simulink model "altitude_controller"  (R2025b)
settings: Solver=FixedStepAuto  StartTime=0.0  StopTime=inf  FixedStep=0.1  RelTol=1e-3
libraries: slpidlib x3, instrumentlib x2, uavutilslib x1
settings Model: Creator=Rakshan  LastModifiedBy=Rakshan

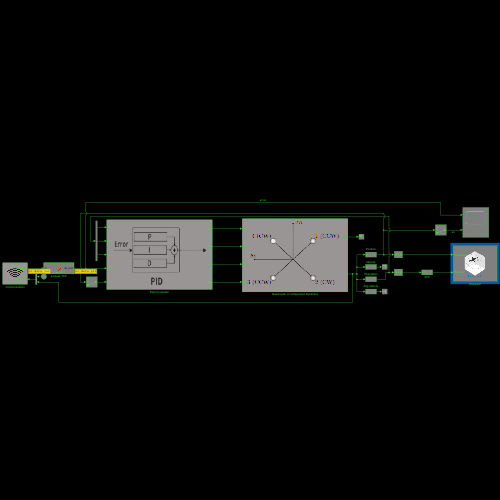
[thumbnail: Simulink's stored preview of the top-level diagram]
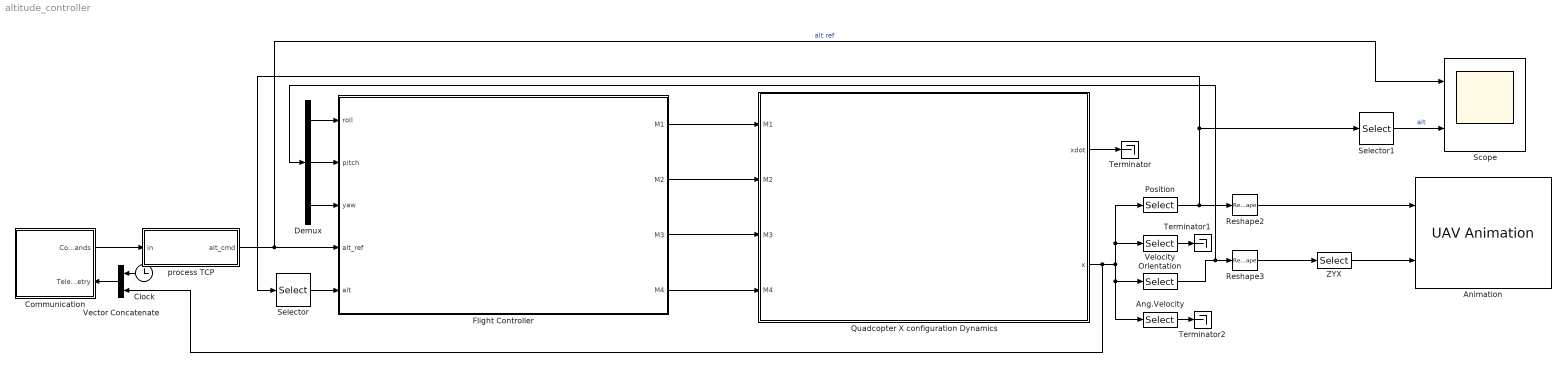
== system altitude_controller ==
  Ang.Velocity : Selector  InputPortWidth=12  IndexOptions=Index vector (dialog)  Indices=[10 11 12]  OutputSizes=1
  Animation : uavutilslib/UAV Animation  NumUAV=1  DynamicUAVConfig=off  UAVType=Multirotor  UAVSize=1  UAVColor=[1, 0.8, 0]  UAVTrajectoryAlpha=1  InertialZDirection=Up  RotationFormat=Euler ZYX  DrawMarkers=off  SampleTime=-1
  Clock : Clock
  Communication : Subsystem
      settings: PortSchema="{\"entries\":[{\"content\":{\"sides\":[{\"content\":{},\"type\":\"ConnectorPlacement.EquallySpacedRectSide\",\"uuid\":\"c4d22659-2383-4074-b14f-30b672d720eb\"},{\"content\":{\"connectorIds\":[\"Out1\",\"In1\"],\"side\":\"RIGHT\"},\"type\":\"ConnectorPlacement.EquallySpacedRectSide\",\"uuid\":\"ba8f1d3a-a611-4235-8c7a-b63cea4c0df4\"},{\"content\":{\"side\":\"TOP\"},\"type\":\"ConnectorPlacement.EquallySpacedRectSide\",\"uuid\":\"69655158-725a-45bc-a08c-7abd09db6858\"}]},\"type\":\"ConnectorPlacement.EquallySpacedConnector\",\"uuid\":\"62f793ea-cbc8-4bf1-b4ec-cf6c7e8acac7\"}],\"packageUris\":[\"http://schema.mathworks.com/mf0/Connector/R2020b\"],\"version\":\"1.0\"}"
      mask Display: image('communication-Photoroom.png');
  Demux : Demux  Outputs=3
  Flight Controller : Subsystem
      mask Display: image('pid-Photoroom.png');
  Orientation : Selector  InputPortWidth=12  IndexOptions=Index vector (dialog)  Indices=[7 8 9]  OutputSizes=1
  Position : Selector  InputPortWidth=12  IndexOptions=Index vector (dialog)  Indices=[1 2 3]  OutputSizes=1
  Quadcopter X configuration Dynamics : Subsystem
      mask Display: image('axis-Photoroom.png');
  Reshape2 : Reshape  OutputDimensionality=Row vector (2-D)
  Reshape3 : Reshape  OutputDimensionality=Row vector (2-D)
  Scope : Scope  NumInputPorts=2
      settings: ActiveDisplayYMinimum=-3.2874736842437113  ActiveDisplayYMaximum=28.143052631582634
  Selector : Selector  InputPortWidth=3  IndexOptions=Index vector (dialog)  Indices=3  OutputSizes=1
  Selector1 : Selector  InputPortWidth=3  IndexOptions=Index vector (dialog)  Indices=3  OutputSizes=1
  Terminator : Terminator
  Terminator1 : Terminator
  Terminator2 : Terminator
  Vector Concatenate : Concatenate
  Velocity : Selector  InputPortWidth=12  IndexOptions=Index vector (dialog)  Indices=[4 5 6]  OutputSizes=1
  ZYX : Selector  InputPortWidth=3  IndexOptions=Index vector (dialog)  Indices=[3 2 1]  OutputSizes=1
  process TCP : MATLAB Function  TreatAsAtomicUnit=on
  wires:
  Communication/1(Commands) -> process TCP/1(in)
  Flight Controller/2(M2) -> Quadcopter X configuration Dynamics/2(M2)
  Flight Controller/1(M1) -> Quadcopter X configuration Dynamics/1(M1)
  Flight Controller/3(M3) -> Quadcopter X configuration Dynamics/3(M3)
  Flight Controller/4(M4) -> Quadcopter X configuration Dynamics/4(M4)
  Quadcopter X configuration Dynamics/1(xdot) -> Terminator/1
  Position/1 -> Selector1/1, Selector/1, Reshape2/1
  Orientation/1 -> Demux/1, Reshape3/1
  Velocity/1 -> Terminator1/1
  Ang.Velocity/1 -> Terminator2/1
  Reshape2/1 -> Animation/1
  Reshape3/1 -> ZYX/1
  ZYX/1 -> Animation/2
  process TCP/1(alt_cmd) -> Scope/1, Flight Controller/4(alt_ref)  "alt ref"
  Demux/1 -> Flight Controller/1(roll)
  Demux/2 -> Flight Controller/2(pitch)
  Demux/3 -> Flight Controller/3(yaw)
  Selector/1 -> Flight Controller/5(alt)
  Selector1/1 -> Scope/2  "alt"
  Quadcopter X configuration Dynamics/2(x) -> Vector Concatenate/2, Orientation/1, Ang.Velocity/1, Position/1, Velocity/1
  Clock/1 -> Vector Concatenate/1
  Vector Concatenate/1 -> Communication/1(Telemetry)

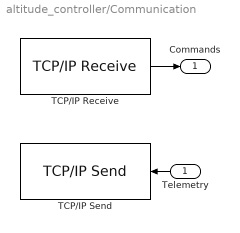
== system altitude_controller/Communication ==
  Telemetry : Inport
  TCP/IP Receive : instrumentlib/TCP//IP Receive  Host=127.0.0.1  Port=55000  DataSize=[ 1, 2 ]  DataType=double  ASCIIFormatting=%f  Terminator=LF  CustomTerminator=10  ByteOrder=big-endian  EnableBlockingMode=on  Timeout=1  SampleTime=0.1  SimulateUsing=Interpreted execution
  TCP/IP Send : instrumentlib/TCP//IP Send  Host=127.0.0.1  Port=55001  ByteOrder=big-endian  EnableBlockingMode=off  Timeout=10  TransferDelay=on  SimulateUsing=Interpreted execution
  Commands : Outport
  wires:
  TCP/IP Receive/1 -> Commands/1
  Telemetry/1 -> TCP/IP Send/1

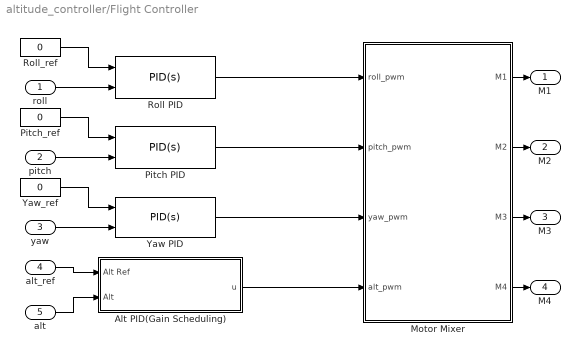
== system altitude_controller/Flight Controller ==
  roll : Inport
  pitch : Inport  Port=2
  yaw : Inport  Port=3
  alt_ref : Inport  Port=4
  alt : Inport  Port=5
  Alt PID(Gain Scheduling) : Subsystem
  Motor Mixer : MATLAB Function  TreatAsAtomicUnit=on
  Pitch PID : slpidlib/PID Controller (2DOF)  Controller=PID  Form=Parallel  TimeDomain=Continuous-time  UseExternalTs=off  SampleTime=-1  IntegratorMethod=Forward Euler  FilterMethod=Forward Euler  ControllerParametersSource=internal  P=1  I=0  UseKiTs=off  D=0  UseExternalDerivativeSource=off  N=100  UseFilter=on  b=1  c=1  TunerSelectOption=Transfer Function Based (PID Tuner App)  InitialConditionSource=internal  InitialConditionForIntegrator=0  InitialConditionForFilter=0  DifferentiatorICPrevScaledInput=0  ExternalReset=none  TrackingMode=off  Kt=1  LimitOutput=off  SatLimitsSource=internal  UpperSaturationLimit=inf  LowerSaturationLimit=-inf  LinearizeAsGain=on  AntiWindupMode=none  Kb=1  LimitIntegrator=off  UpperIntegratorSaturationLimit=inf  LowerIntegratorSaturationLimit=-inf  POutMin=[]  POutMax=[]  IOutMin=[]  IOutMax=[]  DOutMin=[]  DOutMax=[]  NOutMin=[]  NOutMax=[]  bOutMin=[]  bOutMax=[]  cOutMin=[]  cOutMax=[]  SumOutMin=[]  SumOutMax=[]  SaturationOutMin=[]  SaturationOutMax=[]  PParamMin=[]  PParamMax=[]  IParamMin=[]  IParamMax=[]  DParamMin=[]  DParamMax=[]  NParamMin=[]  NParamMax=[]  bParamMin=[]  bParamMax=[]  cParamMin=[]  cParamMax=[]  KbParamMin=[]  KbParamMax=[]  KtParamMin=[]  KtParamMax=[]  KbOutMin=[]  KbOutMax=[]  KtOutMin=[]  KtOutMax=[]  IntegratorOutMin=[]  IntegratorOutMax=[]  FilterOutMin=[]  FilterOutMax=[]  SumI1OutMin=[]  SumI1OutMax=[]  SumI2OutMin=[]  SumI2OutMax=[]  SumI3OutMin=[]  SumI3OutMax=[]  SumI4OutMin=[]  SumI4OutMax=[]  SumDOutMin=[]  SumDOutMax=[]  Sum1OutMin=[]  Sum1OutMax=[]  Sum2OutMin=[]  Sum2OutMax=[]  Sum3OutMin=[]  Sum3OutMax=[]  DifferentiatorOutMin=[]  DifferentiatorOutMax=[]  FilterDiffOutCoefMin=[]  FilterDiffOutCoefMax=[]  ReciprocalOutMin=[]  ReciprocalOutMax=[]  SumDenOutMin=[]  SumDenOutMax=[]  SumNumOutMin=[]  SumNumOutMax=[]  DivideOutMin=[]  DivideOutMax=[]  UdiffTsProdOutMin=[]  UdiffTsProdOutMax=[]  NTsProdOutMin=[]  NTsProdOutMax=[]  UintegralTsProdOutMin=[]  UintegralTsProdOutMax=[]  UngainTsProdOutMin=[]  UngainTsProdOutMax=[]  ClampingZeroOutDataTypeStr=Inherit: Inherit via back propagation  ClampingZeroOutMin=[]  ClampingZeroOutMax=[]  FilterDenConstantOutDataTypeStr=Inherit: Inherit via back propagation  FilterDenConstantOutMin=[]  FilterDenConstantOutMax=[]  PCopyOutDataTypeStr=Inherit: Inherit via back propagation  PCopyOutMin=[]  PCopyOutMax=[]  NCopyOutDataTypeStr=Inherit: Inherit via back propagation  NCopyOutMin=[]  NCopyOutMax=[]  IntegratorContinuousStateAttributes=''  IntegratorStateMustResolveToSignalObject=off  IntegratorRTWStateStorageClass=Auto  FilterContinuousStateAttributes=''  FilterStateMustResolveToSignalObject=off  FilterRTWStateStorageClass=Auto  ParallelPVariant=InternalParameters  IdealPVariant=Disabled  IVariant=InternalParameters  DVariant=InternalParameters  bVariant=InternalParameters  cVariant=InternalParameters  IntegratorVariant=Continuous  SatVariant=Disabled  AWVariant=Passthrough  PCopyVariant=Disabled  TRVariant=Disabled  FdbkBlocksVariant=Forward  IdealPFdbkVariant=Disabled  SatFdbkVariant=Disabled  DerivativeFilterVariant=ContFilter  NVariant=InternalParameters  NCopyVariant=Disabled  FilterICVariant=InternalICsFilter  IntegratorICVariant=InternalICs  ExternalResetVariant=Disabled  TRSumVariant=Passthrough  SumFdbkVariant=Disabled  SumVariant=Sum_PID  TsampFilterVariant=InternalTs  TsampNgainVariant=Passthrough  TsampIntegralVariant=Disabled_SignalSpec  ExternalSaturationOutDataTypeStr=Inherit: Same as second input  DerivativeSourceVariant=ErrorSignal  PreIntVariant=InternalPreInt
  Pitch_ref : Constant  Value=0
  Roll PID : slpidlib/PID Controller (2DOF)  Controller=PID  Form=Parallel  TimeDomain=Continuous-time  UseExternalTs=off  SampleTime=-1  IntegratorMethod=Forward Euler  FilterMethod=Forward Euler  ControllerParametersSource=internal  P=1  I=0  UseKiTs=off  D=0.1  UseExternalDerivativeSource=off  N=100  UseFilter=on  b=1  c=1  TunerSelectOption=Transfer Function Based (PID Tuner App)  InitialConditionSource=internal  InitialConditionForIntegrator=0  InitialConditionForFilter=0  DifferentiatorICPrevScaledInput=0  ExternalReset=none  TrackingMode=off  Kt=1  LimitOutput=off  SatLimitsSource=internal  UpperSaturationLimit=inf  LowerSaturationLimit=-inf  LinearizeAsGain=on  AntiWindupMode=none  Kb=1  LimitIntegrator=off  UpperIntegratorSaturationLimit=inf  LowerIntegratorSaturationLimit=-inf  POutMin=[]  POutMax=[]  IOutMin=[]  IOutMax=[]  DOutMin=[]  DOutMax=[]  NOutMin=[]  NOutMax=[]  bOutMin=[]  bOutMax=[]  cOutMin=[]  cOutMax=[]  SumOutMin=[]  SumOutMax=[]  SaturationOutMin=[]  SaturationOutMax=[]  PParamMin=[]  PParamMax=[]  IParamMin=[]  IParamMax=[]  DParamMin=[]  DParamMax=[]  NParamMin=[]  NParamMax=[]  bParamMin=[]  bParamMax=[]  cParamMin=[]  cParamMax=[]  KbParamMin=[]  KbParamMax=[]  KtParamMin=[]  KtParamMax=[]  KbOutMin=[]  KbOutMax=[]  KtOutMin=[]  KtOutMax=[]  IntegratorOutMin=[]  IntegratorOutMax=[]  FilterOutMin=[]  FilterOutMax=[]  SumI1OutMin=[]  SumI1OutMax=[]  SumI2OutMin=[]  SumI2OutMax=[]  SumI3OutMin=[]  SumI3OutMax=[]  SumI4OutMin=[]  SumI4OutMax=[]  SumDOutMin=[]  SumDOutMax=[]  Sum1OutMin=[]  Sum1OutMax=[]  Sum2OutMin=[]  Sum2OutMax=[]  Sum3OutMin=[]  Sum3OutMax=[]  DifferentiatorOutMin=[]  DifferentiatorOutMax=[]  FilterDiffOutCoefMin=[]  FilterDiffOutCoefMax=[]  ReciprocalOutMin=[]  ReciprocalOutMax=[]  SumDenOutMin=[]  SumDenOutMax=[]  SumNumOutMin=[]  SumNumOutMax=[]  DivideOutMin=[]  DivideOutMax=[]  UdiffTsProdOutMin=[]  UdiffTsProdOutMax=[]  NTsProdOutMin=[]  NTsProdOutMax=[]  UintegralTsProdOutMin=[]  UintegralTsProdOutMax=[]  UngainTsProdOutMin=[]  UngainTsProdOutMax=[]  ClampingZeroOutDataTypeStr=Inherit: Inherit via back propagation  ClampingZeroOutMin=[]  ClampingZeroOutMax=[]  FilterDenConstantOutDataTypeStr=Inherit: Inherit via back propagation  FilterDenConstantOutMin=[]  FilterDenConstantOutMax=[]  PCopyOutDataTypeStr=Inherit: Inherit via back propagation  PCopyOutMin=[]  PCopyOutMax=[]  NCopyOutDataTypeStr=Inherit: Inherit via back propagation  NCopyOutMin=[]  NCopyOutMax=[]  IntegratorContinuousStateAttributes=''  IntegratorStateMustResolveToSignalObject=off  IntegratorRTWStateStorageClass=Auto  FilterContinuousStateAttributes=''  FilterStateMustResolveToSignalObject=off  FilterRTWStateStorageClass=Auto  ParallelPVariant=InternalParameters  IdealPVariant=Disabled  IVariant=InternalParameters  DVariant=InternalParameters  bVariant=InternalParameters  cVariant=InternalParameters  IntegratorVariant=Continuous  SatVariant=Disabled  AWVariant=Passthrough  PCopyVariant=Disabled  TRVariant=Disabled  FdbkBlocksVariant=Forward  IdealPFdbkVariant=Disabled  SatFdbkVariant=Disabled  DerivativeFilterVariant=ContFilter  NVariant=InternalParameters  NCopyVariant=Disabled  FilterICVariant=InternalICsFilter  IntegratorICVariant=InternalICs  ExternalResetVariant=Disabled  TRSumVariant=Passthrough  SumFdbkVariant=Disabled  SumVariant=Sum_PID  TsampFilterVariant=InternalTs  TsampNgainVariant=Passthrough  TsampIntegralVariant=Disabled_SignalSpec  ExternalSaturationOutDataTypeStr=Inherit: Same as second input  DerivativeSourceVariant=ErrorSignal  PreIntVariant=InternalPreInt
  Roll_ref : Constant  Value=0
  Yaw PID : slpidlib/PID Controller (2DOF)  Controller=PID  Form=Parallel  TimeDomain=Continuous-time  UseExternalTs=off  SampleTime=-1  IntegratorMethod=Forward Euler  FilterMethod=Forward Euler  ControllerParametersSource=internal  P=1  I=0  UseKiTs=off  D=0  UseExternalDerivativeSource=off  N=100  UseFilter=on  b=1  c=1  TunerSelectOption=Transfer Function Based (PID Tuner App)  InitialConditionSource=internal  InitialConditionForIntegrator=0  InitialConditionForFilter=0  DifferentiatorICPrevScaledInput=0  ExternalReset=none  TrackingMode=off  Kt=1  LimitOutput=off  SatLimitsSource=internal  UpperSaturationLimit=inf  LowerSaturationLimit=-inf  LinearizeAsGain=on  AntiWindupMode=none  Kb=1  LimitIntegrator=off  UpperIntegratorSaturationLimit=inf  LowerIntegratorSaturationLimit=-inf  POutMin=[]  POutMax=[]  IOutMin=[]  IOutMax=[]  DOutMin=[]  DOutMax=[]  NOutMin=[]  NOutMax=[]  bOutMin=[]  bOutMax=[]  cOutMin=[]  cOutMax=[]  SumOutMin=[]  SumOutMax=[]  SaturationOutMin=[]  SaturationOutMax=[]  PParamMin=[]  PParamMax=[]  IParamMin=[]  IParamMax=[]  DParamMin=[]  DParamMax=[]  NParamMin=[]  NParamMax=[]  bParamMin=[]  bParamMax=[]  cParamMin=[]  cParamMax=[]  KbParamMin=[]  KbParamMax=[]  KtParamMin=[]  KtParamMax=[]  KbOutMin=[]  KbOutMax=[]  KtOutMin=[]  KtOutMax=[]  IntegratorOutMin=[]  IntegratorOutMax=[]  FilterOutMin=[]  FilterOutMax=[]  SumI1OutMin=[]  SumI1OutMax=[]  SumI2OutMin=[]  SumI2OutMax=[]  SumI3OutMin=[]  SumI3OutMax=[]  SumI4OutMin=[]  SumI4OutMax=[]  SumDOutMin=[]  SumDOutMax=[]  Sum1OutMin=[]  Sum1OutMax=[]  Sum2OutMin=[]  Sum2OutMax=[]  Sum3OutMin=[]  Sum3OutMax=[]  DifferentiatorOutMin=[]  DifferentiatorOutMax=[]  FilterDiffOutCoefMin=[]  FilterDiffOutCoefMax=[]  ReciprocalOutMin=[]  ReciprocalOutMax=[]  SumDenOutMin=[]  SumDenOutMax=[]  SumNumOutMin=[]  SumNumOutMax=[]  DivideOutMin=[]  DivideOutMax=[]  UdiffTsProdOutMin=[]  UdiffTsProdOutMax=[]  NTsProdOutMin=[]  NTsProdOutMax=[]  UintegralTsProdOutMin=[]  UintegralTsProdOutMax=[]  UngainTsProdOutMin=[]  UngainTsProdOutMax=[]  ClampingZeroOutDataTypeStr=Inherit: Inherit via back propagation  ClampingZeroOutMin=[]  ClampingZeroOutMax=[]  FilterDenConstantOutDataTypeStr=Inherit: Inherit via back propagation  FilterDenConstantOutMin=[]  FilterDenConstantOutMax=[]  PCopyOutDataTypeStr=Inherit: Inherit via back propagation  PCopyOutMin=[]  PCopyOutMax=[]  NCopyOutDataTypeStr=Inherit: Inherit via back propagation  NCopyOutMin=[]  NCopyOutMax=[]  IntegratorContinuousStateAttributes=''  IntegratorStateMustResolveToSignalObject=off  IntegratorRTWStateStorageClass=Auto  FilterContinuousStateAttributes=''  FilterStateMustResolveToSignalObject=off  FilterRTWStateStorageClass=Auto  ParallelPVariant=InternalParameters  IdealPVariant=Disabled  IVariant=InternalParameters  DVariant=InternalParameters  bVariant=InternalParameters  cVariant=InternalParameters  IntegratorVariant=Continuous  SatVariant=Disabled  AWVariant=Passthrough  PCopyVariant=Disabled  TRVariant=Disabled  FdbkBlocksVariant=Forward  IdealPFdbkVariant=Disabled  SatFdbkVariant=Disabled  DerivativeFilterVariant=ContFilter  NVariant=InternalParameters  NCopyVariant=Disabled  FilterICVariant=InternalICsFilter  IntegratorICVariant=InternalICs  ExternalResetVariant=Disabled  TRSumVariant=Passthrough  SumFdbkVariant=Disabled  SumVariant=Sum_PID  TsampFilterVariant=InternalTs  TsampNgainVariant=Passthrough  TsampIntegralVariant=Disabled_SignalSpec  ExternalSaturationOutDataTypeStr=Inherit: Same as second input  DerivativeSourceVariant=ErrorSignal  PreIntVariant=InternalPreInt
  Yaw_ref : Constant  Value=0
  M1 : Outport
  M2 : Outport  Port=2
  M3 : Outport  Port=3
  M4 : Outport  Port=4
  wires:
  pitch/1 -> Pitch PID/2
  Roll PID/1 -> Motor Mixer/1(roll_pwm)
  Pitch_ref/1 -> Pitch PID/1
  Pitch PID/1 -> Motor Mixer/2(pitch_pwm)
  Roll_ref/1 -> Roll PID/1
  yaw/1 -> Yaw PID/2
  Yaw_ref/1 -> Yaw PID/1
  Yaw PID/1 -> Motor Mixer/3(yaw_pwm)
  Motor Mixer/3(M3) -> M3/1
  roll/1 -> Roll PID/2
  Motor Mixer/2(M2) -> M2/1
  Motor Mixer/1(M1) -> M1/1
  Motor Mixer/4(M4) -> M4/1
  alt_ref/1 -> Alt PID(Gain Scheduling)/1(Alt Ref)
  alt/1 -> Alt PID(Gain Scheduling)/2(Alt)
  Alt PID(Gain Scheduling)/1(u) -> Motor Mixer/4(alt_pwm)

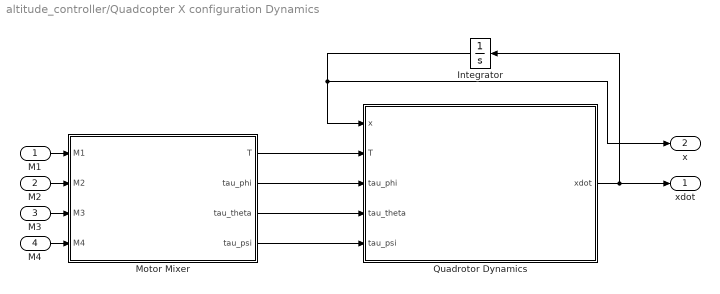
== system altitude_controller/Quadcopter X configuration Dynamics ==
  M1 : Inport
  M2 : Inport  Port=2
  M3 : Inport  Port=3
  M4 : Inport  Port=4
  Integrator : Integrator
  Motor Mixer : MATLAB Function  TreatAsAtomicUnit=on
  Quadrotor Dynamics : MATLAB Function  TreatAsAtomicUnit=on
  xdot : Outport
  x : Outport  Port=2
  wires:
  Quadrotor Dynamics/1(xdot) -> xdot/1, Integrator/1
  Motor Mixer/4(tau_psi) -> Quadrotor Dynamics/5(tau_psi)
  Motor Mixer/2(tau_phi) -> Quadrotor Dynamics/3(tau_phi)
  M2/1 -> Motor Mixer/2(M2)
  Motor Mixer/1(T) -> Quadrotor Dynamics/2(T)
  M3/1 -> Motor Mixer/3(M3)
  Motor Mixer/3(tau_theta) -> Quadrotor Dynamics/4(tau_theta)
  M1/1 -> Motor Mixer/1(M1)
  M4/1 -> Motor Mixer/4(M4)
  Integrator/1 -> x/1, Quadrotor Dynamics/1(x)

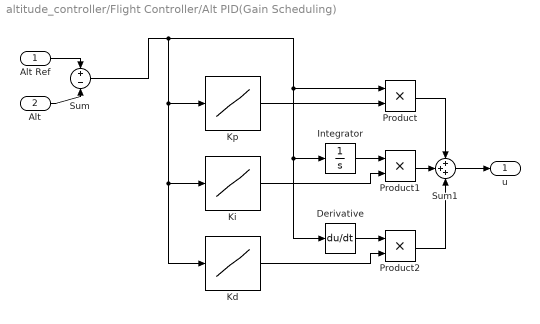
== system altitude_controller/Flight Controller/Alt PID(Gain Scheduling) ==
  Alt Ref : Inport
  Alt : Inport  Port=2
  Derivative : Derivative
  Integrator : Integrator
  Kd : Lookup_n-D  NumberOfTableDimensions=1  BreakpointsForDimension1=[0;10;20;30;40;50]  Table=[130; 125; 120; 112; 110; 106]  InternalRulePriority=Speed  RndMeth=Simplest
  Ki : Lookup_n-D  NumberOfTableDimensions=1  BreakpointsForDimension1=[0;10;20;30;40;50]  Table=[8; 7; 6; 5; 4; 3]  InternalRulePriority=Speed  RndMeth=Simplest
  Kp : Lookup_n-D  NumberOfTableDimensions=1  BreakpointsForDimension1=[0;10;20;30;40;50]  Table=[70; 65; 60; 48; 32; 15]  InternalRulePriority=Speed  RndMeth=Simplest
  Product : Product
  Product1 : Product
  Product2 : Product
  Sum : Sum  Inputs=+|-
  Sum1 : Sum  Inputs=+++
  u : Outport
  wires:
  Product/1 -> Sum1/1
  Sum/1 -> Kd/1, Ki/1, Kp/1, Product/1, Derivative/1, Integrator/1
  Derivative/1 -> Product2/1
  Product2/1 -> Sum1/3
  Alt Ref/1 -> Sum/1
  Ki/1 -> Product1/2
  Kd/1 -> Product2/2
  Kp/1 -> Product/2
  Integrator/1 -> Product1/1
  Product1/1 -> Sum1/2
  Alt/1 -> Sum/2
  Sum1/1 -> u/1

== matlab function altitude_controller/process TCP ==
  data: in input; alt_cmd output
function alt_cmd = processTCP(in)
%#codegen
% in: [start_flag, altitude_value]
% Output:
%   alt_cmd - held altitude command (changes only when input altitude changes)

persistent alt_hold prev_alt
if isempty(alt_hold)
    alt_hold = 0;
    prev_alt = -9999; % impossible initial value
end

start_flag = in(1);
alt_value  = in(2);

if start_flag == 1
    % latch only if altitude value changes
    if alt_value ~= prev_alt
        alt_hold = alt_value;
        prev_alt = alt_value;
    end
end

% hold altitude if start_flag = 0
alt_cmd = alt_hold;

== matlab function altitude_controller/Flight Controller/Motor Mixer ==
  data: roll_pwm input; M1 output; pitch_pwm input; yaw_pwm input; alt_pwm input; M2 output; M3 output; M4 output
function [M1, M2, M3, M4] = motorMixerENU(roll_pwm, pitch_pwm, yaw_pwm, alt_pwm)
%#codegen
% Quadcopter Motor Mixer (ENU Frame)
% Configuration based on provided diagram:
%   M1 - Front Left (CW)
%   M2 - Rear Left (CCW)
%   M3 - Front Right (CCW)
%   M4 - Rear Right (CW)

% --- Mixer equations ---
M1 = 1000+alt_pwm - pitch_pwm - roll_pwm - yaw_pwm; % Front Left (CW)
M2 = 1000+alt_pwm + pitch_pwm - roll_pwm + yaw_pwm; % Rear Left (CCW)
M3 = 1000+alt_pwm - pitch_pwm + roll_pwm + yaw_pwm; % Front Right (CCW)
M4 = 1000+alt_pwm + pitch_pwm + roll_pwm - yaw_pwm; % Rear Right (CW)

% --- Optional saturation for PWM limits ---
M1 = max(min(M1, 2000), 1000);
M2 = max(min(M2, 2000), 1000);
M3 = max(min(M3, 2000), 1000);
M4 = max(min(M4, 2000), 1000);
end

== matlab function altitude_controller/Quadcopter X configuration Dynamics/Motor Mixer ==
  data: M1 input; T output; tau_phi output; M2 input; M3 input; M4 input; tau_theta output; tau_psi output
function [T, tau_phi, tau_theta, tau_psi] = MotorMix(M1, M2, M3, M4)
%#codegen
% MotorMix: Converts motor PWM inputs (M1–M4) to total thrust and torques
%
% Inputs:
%   M1–M4 : Motor PWM signals [1000, 2000]
%
% Outputs:
%   T          : Total thrust (N)
%   tau_phi    : Roll torque (Nm)
%   tau_theta  : Pitch torque (Nm)
%   tau_psi    : Yaw torque (Nm)

%% --- Parameters ---
Tmax = 10;      % Example max thrust per motor (N) at full input
L = 0.25;       % Arm length (m)
kq = 0.01;      % Yaw moment coefficient

% Derived constant
kT = Tmax;      % Thrust coefficient from document
r = L / sqrt(2);

%% --- Normalize PWM to control input (Eq. 3) ---
u1 = min(max((M1 - 1000)/1000, 0), 1);
u2 = min(max((M2 - 1000)/1000, 0), 1);
u3 = min(max((M3 - 1000)/1000, 0), 1);
u4 = min(max((M4 - 1000)/1000, 0), 1);

%% --- Compute individual motor thrusts (Eq. 4) ---
T1 = kT * u1^2;
T2 = kT * u2^2;
T3 = kT * u3^2;
T4 = kT * u4^2;

%% --- Total Thrust and Torques ---
T        = T1 + T2 + T3 + T4;                          % Eq. (5)
tau_phi  = r * (-T1 - T2 + T3 + T4);                   % Eq. (6)
tau_theta= r * (-T1 + T2 + T3 - T4);                   % Eq. (7)
tau_psi  = kq * (T1 - T2 + T3 - T4);                   % Eq. (8)
end

== matlab function altitude_controller/Quadcopter X configuration Dynamics/Quadrotor Dynamics ==
  data: x input; xdot output; T input; tau_phi input; tau_theta input; tau_psi input
function xdot = QuadrotorDynamics(x, T, tau_phi, tau_theta, tau_psi)
%#codegen
% QuadrotorDynamics: Computes nonlinear state derivatives xdot = f(x,u)
% with simple ground contact model (z >= 0).
%
% Inputs:
%   x  = [x y z xdot ydot zdot phi theta psi p q r]'
%   T  = total thrust (N)
%   tau_phi, tau_theta, tau_psi = body torques (Nm)
%
% Output:
%   xdot = [xdot ydot zdot xddot yddot zddot phidot thetadot psidot pdot qdot rdot]'

%% --- Parameters ---
m  = 1;       % mass (kg)
g  = 9.81;    % gravity (m/s^2)
Ix = 0.02;    % inertia around x (kg·m^2)
Iy = 0.02;    % inertia around y (kg·m^2)
Iz = 0.04;    % inertia around z (kg·m^2)

%% --- Extract states ---
xpos  = x(1);  ypos  = x(2);  zpos = x(3);
xd    = x(4);  yd    = x(5);  zd   = x(6);
phi   = x(7);  theta = x(8);  psi  = x(9);
p     = x(10); q     = x(11); r    = x(12);

%% --- Rotation matrix (Body → Inertial), Eq. (11) ---
cphi = cos(phi); sphi = sin(phi);
cth  = cos(theta); sth = sin(theta);
cpsi = cos(psi); spsi = sin(psi);

R = [ cth*cpsi, sphi*sth*cpsi - cphi*spsi, cphi*sth*cpsi + sphi*spsi;
      cth*spsi, sphi*sth*spsi + cphi*cpsi, cphi*sth*spsi - sphi*cpsi;
     -sth,      sphi*cth,                 cphi*cth];

%% --- Translational accelerations (Eq. 12) ---
acc = (1/m) * (R * [0;0;T]) - [0;0;g];
xdd = acc(1);
ydd = acc(2);
zdd = acc(3);

%% --- Angular rate dynamics (Eq. 14) ---
pdot = ((Iy - Iz)/Ix) * q * r + tau_phi / Ix;
qdot = ((Iz - Ix)/Iy) * r * p + tau_theta / Iy;
rdot = ((Ix - Iy)/Iz) * p * q + tau_psi / Iz;

%% --- Euler angle kinematics (Eq. 15–16) ---
TTheta = [1, sin(phi)*tan(theta),  cos(phi)*tan(theta);
          0, cos(phi),            -sin(phi);
          0, sin(phi)/cos(theta),  cos(phi)/cos(theta)];
angdot = TTheta * [p; q; r];
phidot   = angdot(1);
thetadot = angdot(2);
psidot   = angdot(3);

%% --- Assemble preliminary state derivatives ---
xdot = [ xd; yd; zd; xdd; ydd; zdd; phidot; thetadot; psidot; pdot; qdot; rdot ];

%% --- Ground contact logic: enforce z >= 0 ---
eps = 1e-6; % small tolerance to avoid chattering
% xdot(3) is z_dot (vertical velocity), xdot(6) is z_ddot (vertical accel)
if zpos <= eps && xdot(3) <= 0
    % On or below ground and moving (or about to move) downward:
    % - Prevent further downward motion (no negative z_dot)
    % - Block downward acceleration, allow upward acceleration to enable takeoff
    xdot(3) = 0;                % freeze vertical velocity (no downward movement)
    xdot(6) = max(xdot(6), 0);  % allow positive accel (takeoff), block negative accel
end

end
